simulink model "FINALFILE2025"  (R2024b)
settings: Solver=VariableStepAuto  StartTime=0.0  StopTime=1  RelTol=1e-3
libraries: spsIGBTDiodeLib x6, spsVoltageMeasurementLib x3, spsTriangleGeneratorLib x3, spsDCVoltageSourceLib x1, spsPermanentMagnetSynchronousMachineLib x1, sps_lib x1
settings Model: Creator=ahmedmajid  LastModifiedBy=ahmedmajid

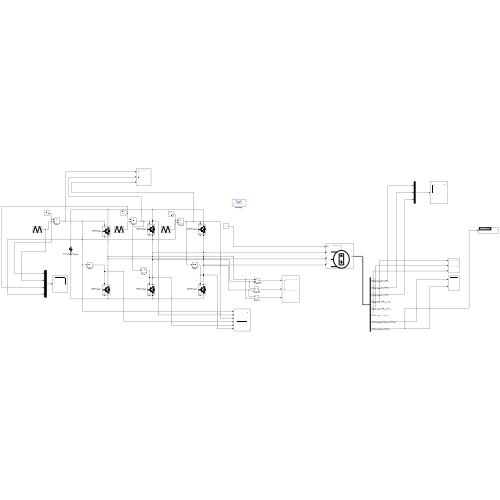
[thumbnail: Simulink's stored preview of the top-level diagram]
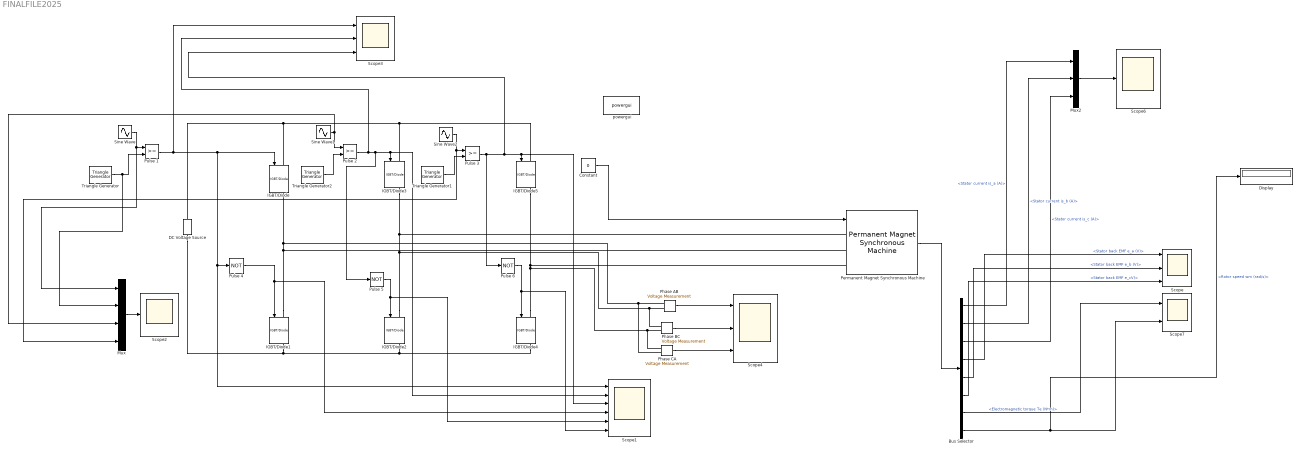
== system FINALFILE2025 ==
  Bus Selector : BusSelector  OutputSignals=Stator current is_a (A),Stator current is_b (A),Stator current is_c (A),Stator back EMF e_a (V),Stator back EMF e_b (V),Stator back EMF e_cV),Electromagnetic torque Te (N*m),Rotor speed wm (rad/s)
  Constant : Constant  Value=0
  DC Voltage Source : spsDCVoltageSourceLib/DC Voltage Source  Amplitude=400  Measurements=None
  Display : Display
  IGBT/Diode{,1..5} (6 alike) : spsIGBTDiodeLib/IGBT//Diode  Ron=1e-3  Rs=1e5  Cs=inf  Measurements=on
  Mux : Mux
  Mux2 : Mux  Inputs=3
  Permanent Magnet Synchronous Machine : spsPermanentMagnetSynchronousMachineLib/Permanent Magnet Synchronous Machine  NbPhases=3  FluxDistribution=Trapezoidal  RotorType=Round  MechanicalLoad=Torque Tm  PresetModel="01:  0.8 Nm 300 Vdc 3000 RPM - 0.8 Nm"  ShowDetailedParameters=on  MeasurementBus=off  Resistance=18.7  Inductance=8.5e-3  dqInductances=[8.5e-3,8.5e-3]  La=0.02682  MachineConstant=Flux linkage established by magnets (V.s)  Flux=0.1716  VoltageCst=71.8796  TorqueCst=0.6864  Flat=120  Mechanical=[2.26e-05 1.349e-05 2 0]  PolePairs=2  InitialConditions=[0,0, 0,0]  InitialConditions5ph=[0 0 0 0 0 0]  RefAngle=Aligned with phase A axis (original Park)  IterativeDiscreteModel=Trapezoidal robust  TsBlock=1e-5  TsPowergui=0
  Phase AB : spsVoltageMeasurementLib/Voltage Measurement  PhasorSimulation=off  OutputType=Complex  PSBequivalent=0
  Phase BC : spsVoltageMeasurementLib/Voltage Measurement  PhasorSimulation=off  OutputType=Complex  PSBequivalent=0
  Phase CA : spsVoltageMeasurementLib/Voltage Measurement  PhasorSimulation=off  OutputType=Complex  PSBequivalent=0
  Pulse 1 : RelationalOperator  OutDataTypeStr=boolean  RndMeth=Simplest  InputSameDT=off
  Pulse 2 : RelationalOperator  OutDataTypeStr=boolean  RndMeth=Simplest  InputSameDT=off
  Pulse 3 : RelationalOperator  OutDataTypeStr=boolean  RndMeth=Simplest  InputSameDT=off
  Pulse 4 : Logic  Operator=NOT  AllPortsSameDT=off  OutDataTypeStr=boolean
  Pulse 5 : Logic  Operator=NOT  AllPortsSameDT=off  OutDataTypeStr=boolean
  Pulse 6 : Logic  Operator=NOT  AllPortsSameDT=off  OutDataTypeStr=boolean
  Scope : Scope  NumInputPorts=3
  Scope1 : Scope  NumInputPorts=6
  Scope2 : Scope
  Scope3 : Scope  NumInputPorts=3
  Scope4 : Scope  NumInputPorts=3
  Scope6 : Scope
  Scope7 : Scope  NumInputPorts=2
  Sine Wave : Sin  Frequency=2*pi*50  SampleTime=0
  Sine Wave1 : Sin  Frequency=2*pi*50  Phase=120*(pi/180)  SampleTime=0
  Sine Wave2 : Sin  Frequency=2*pi*50  Phase=240*(pi/180)  SampleTime=0
  Triangle Generator : spsTriangleGeneratorLib/Triangle Generator  Freq=10e3  Phase=0  Ts=0
  Triangle Generator1 : spsTriangleGeneratorLib/Triangle Generator  Freq=50e3  Phase=0  Ts=0
  Triangle Generator2 : spsTriangleGeneratorLib/Triangle Generator  Freq=50e3  Phase=0  Ts=0
  powergui : sps_lib/powergui  Priority=1  SimulationMode=Discrete  SampleTime=1e-6  frequency=60  Iterations=50  frequencyindice=0  Pbase=100e6  ErrMax=1e-4  UnitsV=kV  UnitsW=MW  buscounter=0  FunctionMessages=off  echomessages=off  EnableUseOfTLC=off  CurrentSourceSwitches=off  DisableSnubberDevices=off  DisableRonSwitches=off  DisableVfSwitches=off  DisplayEquations=off  AutomaticDiscreteSolvers=off  SolverType=Tustin/Backward Euler (TBE)  Interpol=off  ExternalGateDelay=off  methode=off  Ts=100  x0status=blocks  SPID=on  SwTol=0  HookPort=off  NonlinearTolerance=1e-4  nMaxIteration=100  ContinueOnMaxIteration=off  RestoreLinks=warning  ResistiveCurrentMeasurement=off  Frange=[0:2:500]  Ylog=off  Xlog=on  ShowGrid=off  save=off  variable=ZData  structure=0  ZoomFFT=off  StartTime=0.0  cycles=1  DisplayStyle=1  fundamental=60  FreqAxis=off  MaxFrequency=1000  frequencyindicesteady=1  RmsSteady=1  display=off
  wires:
  Bus Selector/1 -> Mux2/1  "<Stator current is_a (A)>"
  Permanent Magnet Synchronous Machine/1 -> Bus Selector/1
  Sine Wave/1 -> Mux/1, Pulse 1/1
  Sine Wave2/1 -> Mux/4, Pulse 3/1
  Sine Wave1/1 -> Mux/3, Pulse 2/1
  Pulse 4/1 -> Scope1/4, IGBT/Diode1/1
  Pulse 3/1 -> Scope3/3, Scope1/3, IGBT/Diode5/1, Pulse 6/1
  Pulse 6/1 -> Scope1/6, IGBT/Diode4/1
  Pulse 1/1 -> Scope3/1, Scope1/1, Pulse 4/1, IGBT/Diode/1
  Pulse 2/1 -> Scope3/2, Scope1/2, IGBT/Diode3/1, Pulse 5/1
  Pulse 5/1 -> Scope1/5, IGBT/Diode2/1
  Constant/1 -> Permanent Magnet Synchronous Machine/1
  Triangle Generator/1 -> Mux/2, Pulse 1/2
  Triangle Generator2/1 -> Pulse 2/2
  Triangle Generator1/1 -> Pulse 3/2
  Mux/1 -> Scope2/1
  Phase AB/1 -> Scope4/1
  Phase BC/1 -> Scope4/2
  Phase CA/1 -> Scope4/3
  Mux2/1 -> Scope6/1
  Bus Selector/2 -> Mux2/2  "<Stator current is_b (A)>"
  Bus Selector/3 -> Mux2/3  "<Stator current is_c (A)>"
  Bus Selector/7 -> Scope7/1  "<Electromagnetic torque Te (N*m)>"
  Bus Selector/8 -> Display/1, Scope7/2  "<Rotor speed wm (rad/s)>"
  Bus Selector/4 -> Scope/1  "<Stator back EMF e_a (V)>"
  Bus Selector/5 -> Scope/2  "<Stator back EMF e_b (V)>"
  Bus Selector/6 -> Scope/3  "<Stator back EMF e_cV)>"
  connections:
  IGBT/Diode5/LConn1 -- DC Voltage Source/RConn1 -- IGBT/Diode/LConn1 -- IGBT/Diode3/LConn1
  IGBT/Diode2/LConn1 -- Permanent Magnet Synchronous Machine/LConn1 -- IGBT/Diode3/RConn1 -- Phase BC/LConn1 -- Phase AB/LConn2
  IGBT/Diode4/LConn1 -- IGBT/Diode5/RConn1 -- Permanent Magnet Synchronous Machine/LConn3 -- Phase CA/LConn1 -- Phase BC/LConn2
  IGBT/Diode2/RConn1 -- IGBT/Diode4/RConn1 -- DC Voltage Source/LConn1 -- IGBT/Diode1/RConn1
  IGBT/Diode1/LConn1 -- IGBT/Diode/RConn1 -- Phase CA/LConn2 -- Phase AB/LConn1 -- Permanent Magnet Synchronous Machine/LConn2
